simulink model "model_filters_bandpass"  (R2018a)
settings: Solver=VariableStepAuto  StartTime=0.0  StopTime=6  RelTol=1e-3
PreLoadFcn:
  | load('alberto_data.mat')
model workspace (MAT data in the model file):
  fc = Simulink.Parameter
  fc.Value = 10
  fc.DataType = 'auto'
  fc.Dimensions = [1 1]
undefined symbols (not defined in the file or in its folder): fc_2
libraries: dspmlti4 x1, dsparch4 x1
settings Model: Creator=stefanobuccelli  LastModifiedBy=stefanobuccelli

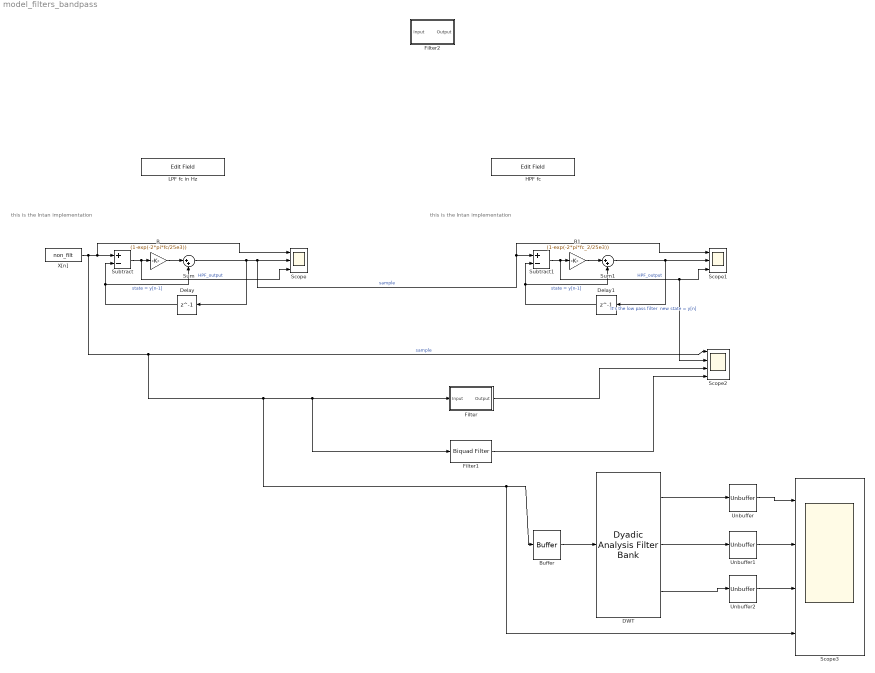
== system model_filters_bandpass ==
  note: this is the Intan implementation
  note: this is the Intan implementation
  B : Gain  Gain=(1-exp(-2*pi*fc/25e3))
  B1 : Gain  Gain=(1-exp(-2*pi*fc_2/25e3))
  Buffer : Buffer  OutputFrames=off
  DWT : dspmlti4/Dyadic Analysis Filter Bank  Wname=Biorthogonal  OrdRec_ordDec=[1 / 1]  Order=4  LPF="[0.0352   -0.0854   -0.1350   0.4599   0.8069   0.3327]"  HPF="[-0.3327    0.8069   -0.4599   -0.1350    0.0854    0.0352]"  NumLevels=2  tree=Asymmetric  Output=Multiple ports  OutputFrames=off
      settings: SourceProductName=DSP System Toolbox  SourceProductBaseCode=DS
  Delay : Delay  DelayLength=1
  Delay1 : Delay  DelayLength=1
  Filter : Subsystem  Tag=FilterWizardSubSystem
      settings: ErrorFcn=dspFilterRealizedInBasicElemsAlgLoopErrFcnCallback
  Filter1 : dsparch4/Biquad Filter  Tag=BlockMethodSubSystem  IIRFiltStruct=Direct form II  CoeffSource=Specify via dialog  BiQuadCoeffs=[1 0 -1 1 -1.99992831176449659 0.999934693355535975;1 0 -1 1 -1.99995897844210879 0.999961229592609468;1 0 -1 1 -1.9997987901469445 0.999805141210744264;1 0 -1 1 -1.99988145168083653 0.999883712729304319;1 0 -1 1 -1.99967234895056767 0.999678637128671221;1 0 -1 1 -1.99980407875227995 0.999806362624380718;1 0 -1 1 -1.99955099756990373 0.999557193946188249;1 0 -1 1 -1.99972693907547727 0.99972925660954115;1 0 -1 1 -1.99943663285096473 0.999442710022172998;1 0 -1 1 -1.99965016883954116 0.9996525313616208;1 0 -1 1 -1.99933100019716337 0.999336932639597553;1 0 -1 1 -1.99957397919015145 0.999576398765119833;1 0 -1 1 -1.9992355440381222 0.999241307193421191;1 0 -1 1 -1.99949878587869789 0.99950127682582135;1 0 -1 1 -1.99915183537296492 0.999157410502061416;1 0 -1 1 -1.99942476285883375 0.999427337308120389;1 0 -1 1 -1.99908090623175538 0.999086276782043647;1 0 -1 1 -1.99935249017064054 0.999355162168056532;1 0 -1 1 -1.99902340207156426 0.999028553701973743;1 0 -1 1 -1.9992827852671633 0.999285571050194887;1 0 -1 1 -1.99897998508968944 0.998984908853462139;1 0 -1 1 -1.99921628495669279 0.999219199786026469;1 0 -1 1 -1.99895111246551194 0.998955805384742823;1 0 -1 1 -1.99915365408997703 0.999156711568302991;1 0 -1 1 -1.99893596859811895 0.998940426918434321;1 0 -1 1 -1.99909664204870818 0.999099860745045421;1 0 -1 1 -1.99893512415378805 0.998939355238140814;1 0 -1 1 -1.99904541432707017 0.999048805016561126;1 0 -1 1 -1.99894631798573164 0.998950322878909391;1 0 -1 1 -1.99900276323179904 0.999006345900247505;1 0 -1 1 -1.99896927984751582 0.998973067828728856]  a0Flag=Warning  IC=0  ICnum=0  ICden=0  denAccumFracLength=30  denProdOutputFracLength=30  secondMemoryFracLength=15  roundingMode=Floor  overflowMode=off  ScaleValues=[0.000513716433989335787;0.000513716433989335787;0.000513689840814086441;0.000513689840814086441;0.000513663661699879275;0.000513663661699879275;0.000513638165030047425;0.000513638165030047425;0.000513613612073675926;0.000513613612073675926;0.000513590254319449798;0.000513590254319449798;0.000513568330913804225;0.000513568330913804225;0.000513548066228893744;0.000513548066228893744;0.000513529667584439208;0.000513529667584439208;0.00051351332314583881;0.00051351332314583881;0.000513499200019070586;0.000513499200019070586;0.000513487442560885479;0.000513487442560885479;0.000513478170920615164;0.000513478170920615164;0.000513471479827616378;0.000513471479827616378;0.000513467437635966185;0.000513467437635966185;0.000513466085635530317;1]  optimizeScaleValues=on  ScaleValueMode=Specify via input port (g)  scaleValueFracLength=14  FilterSource=Specify via dialog  FilterObject=BQF
      settings: SourceProductName=DSP System Toolbox
  Filter2 : Subsystem  Tag=FilterWizardSubSystem
      settings: ErrorFcn=dspFilterRealizedInBasicElemsAlgLoopErrFcnCallback
  HPF fc : EditField  WebBlockId=433  LabelPosition=Hide  Alignment=Center
  LPF fc in Hz : EditField  WebBlockId=206  LabelPosition=Hide  Alignment=Center
  Scope : Scope  NumInputPorts=3
  Scope1 : Scope  NumInputPorts=3
  Scope2 : Scope  NumInputPorts=4
  Scope3 : Scope  NumInputPorts=4
  Subtract : Sum  Inputs=+-
  Subtract1 : Sum  Inputs=+-
  Sum : Sum  Inputs=|++
  Sum1 : Sum  Inputs=|++
  Unbuffer : Unbuffer
  Unbuffer1 : Unbuffer
  Unbuffer2 : Unbuffer
  X[n] : FromWorkspace  VariableName=non_filt  SampleTime=1/25e3  OutputAfterFinalValue=Setting to zero
  wires:
  X[n]/1 -> Scope3/4, Buffer/1, Filter1/1, Filter/1(Input), Scope2/1, Scope/1, Subtract/1  "sample"
  Subtract/1 -> Scope/3, B/1  "HPF_output"
  B/1 -> Sum/1
  Delay/1 -> Sum/2, Subtract/2  "state = y[n-1]"
  Subtract1/1 -> Scope2/2, Scope1/3, B1/1  "HPF_output"
  B1/1 -> Sum1/1
  Delay1/1 -> Sum1/2, Subtract1/2  "state = y[n-1]"
  Sum1/1 -> Delay1/1, Scope1/2  "It's the low pass filter  new state = y[n]"
  Sum/1 -> Delay/1, Scope1/1, Subtract1/1, Scope/2  "sample"
  Filter/1(Output) -> Scope2/3
  Filter1/1 -> Scope2/4
  Buffer/1 -> DWT/1
  Unbuffer/1 -> Scope3/1
  Unbuffer1/1 -> Scope3/2
  Unbuffer2/1 -> Scope3/3
  DWT/2 -> Unbuffer1/1
  DWT/3 -> Unbuffer2/1
  DWT/1 -> Unbuffer/1

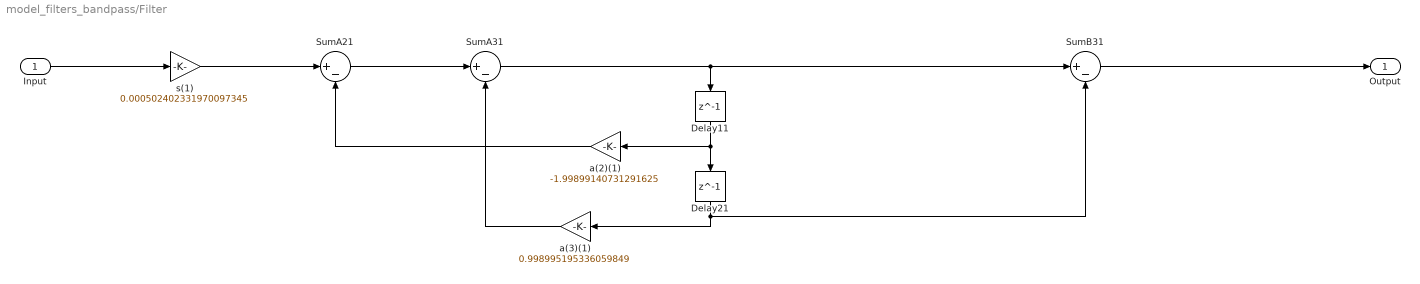
== system model_filters_bandpass/Filter ==
  Input : Inport
  Delay11 : Delay  DelayLength=1  InitialCondition=0
  Delay21 : Delay  DelayLength=1  InitialCondition=0
  SumA21 : Sum  Inputs=|+-  RndMeth=Nearest  SaturateOnIntegerOverflow=on  OutDataTypeStr=Inherit: Same as first input
  SumA31 : Sum  Inputs=|+-  RndMeth=Nearest  SaturateOnIntegerOverflow=on  OutDataTypeStr=Inherit: Same as first input
  SumB31 : Sum  Inputs=|+-  RndMeth=Nearest  SaturateOnIntegerOverflow=on  OutDataTypeStr=Inherit: Same as first input
  a(2)(1) : Gain  Gain=-1.99899140731291625  ParamDataTypeStr=double  RndMeth=Nearest  SaturateOnIntegerOverflow=on  OutDataTypeStr=Inherit: Same as input
  a(3)(1) : Gain  Gain=0.998995195336059849  ParamDataTypeStr=double  RndMeth=Nearest  SaturateOnIntegerOverflow=on  OutDataTypeStr=Inherit: Same as input
  s(1) : Gain  Gain=0.000502402331970097345  ParamDataTypeStr=double  RndMeth=Nearest  SaturateOnIntegerOverflow=on  OutDataTypeStr=Inherit: Same as input
  Output : Outport
  wires:
  Input/1 -> s(1)/1
  s(1)/1 -> SumA21/1
  SumA21/1 -> SumA31/1
  SumA31/1 -> SumB31/1, Delay11/1
  SumB31/1 -> Output/1
  a(2)(1)/1 -> SumA21/2
  Delay11/1 -> a(2)(1)/1, Delay21/1
  a(3)(1)/1 -> SumA31/2
  Delay21/1 -> a(3)(1)/1, SumB31/2

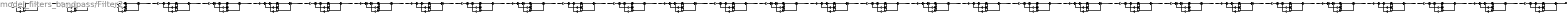
== system model_filters_bandpass/Filter2 ==
  Input : Inport
  Delay{11..19,21..29,110..131,210..231} (62 alike) : Delay  DelayLength=1  InitialCondition=0
  SumA{21..29,31..39,210..231,310..331} (62 alike) : Sum  Inputs=|+-  RndMeth=Nearest  SaturateOnIntegerOverflow=on  OutDataTypeStr=Inherit: Same as first input
  SumB{31..39,310..331} (31 alike) : Sum  Inputs=|+-  RndMeth=Nearest  SaturateOnIntegerOverflow=on  OutDataTypeStr=Inherit: Same as first input
  a(2)(1) : Gain  Gain=-1.99992831176449659  ParamDataTypeStr=double  RndMeth=Nearest  SaturateOnIntegerOverflow=on  OutDataTypeStr=Inherit: Same as input
  a(2)(10) : Gain  Gain=-1.99965016883954116  ParamDataTypeStr=double  RndMeth=Nearest  SaturateOnIntegerOverflow=on  OutDataTypeStr=Inherit: Same as input
  a(2)(11) : Gain  Gain=-1.99933100019716337  ParamDataTypeStr=double  RndMeth=Nearest  SaturateOnIntegerOverflow=on  OutDataTypeStr=Inherit: Same as input
  a(2)(12) : Gain  Gain=-1.99957397919015145  ParamDataTypeStr=double  RndMeth=Nearest  SaturateOnIntegerOverflow=on  OutDataTypeStr=Inherit: Same as input
  a(2)(13) : Gain  Gain=-1.9992355440381222  ParamDataTypeStr=double  RndMeth=Nearest  SaturateOnIntegerOverflow=on  OutDataTypeStr=Inherit: Same as input
  a(2)(14) : Gain  Gain=-1.99949878587869789  ParamDataTypeStr=double  RndMeth=Nearest  SaturateOnIntegerOverflow=on  OutDataTypeStr=Inherit: Same as input
  a(2)(15) : Gain  Gain=-1.99915183537296492  ParamDataTypeStr=double  RndMeth=Nearest  SaturateOnIntegerOverflow=on  OutDataTypeStr=Inherit: Same as input
  a(2)(16) : Gain  Gain=-1.99942476285883375  ParamDataTypeStr=double  RndMeth=Nearest  SaturateOnIntegerOverflow=on  OutDataTypeStr=Inherit: Same as input
  a(2)(17) : Gain  Gain=-1.99908090623175538  ParamDataTypeStr=double  RndMeth=Nearest  SaturateOnIntegerOverflow=on  OutDataTypeStr=Inherit: Same as input
  a(2)(18) : Gain  Gain=-1.99935249017064054  ParamDataTypeStr=double  RndMeth=Nearest  SaturateOnIntegerOverflow=on  OutDataTypeStr=Inherit: Same as input
  a(2)(19) : Gain  Gain=-1.99902340207156426  ParamDataTypeStr=double  RndMeth=Nearest  SaturateOnIntegerOverflow=on  OutDataTypeStr=Inherit: Same as input
  a(2)(2) : Gain  Gain=-1.99995897844210879  ParamDataTypeStr=double  RndMeth=Nearest  SaturateOnIntegerOverflow=on  OutDataTypeStr=Inherit: Same as input
  a(2)(20) : Gain  Gain=-1.9992827852671633  ParamDataTypeStr=double  RndMeth=Nearest  SaturateOnIntegerOverflow=on  OutDataTypeStr=Inherit: Same as input
  a(2)(21) : Gain  Gain=-1.99897998508968944  ParamDataTypeStr=double  RndMeth=Nearest  SaturateOnIntegerOverflow=on  OutDataTypeStr=Inherit: Same as input
  a(2)(22) : Gain  Gain=-1.99921628495669279  ParamDataTypeStr=double  RndMeth=Nearest  SaturateOnIntegerOverflow=on  OutDataTypeStr=Inherit: Same as input
  a(2)(23) : Gain  Gain=-1.99895111246551194  ParamDataTypeStr=double  RndMeth=Nearest  SaturateOnIntegerOverflow=on  OutDataTypeStr=Inherit: Same as input
  a(2)(24) : Gain  Gain=-1.99915365408997703  ParamDataTypeStr=double  RndMeth=Nearest  SaturateOnIntegerOverflow=on  OutDataTypeStr=Inherit: Same as input
  a(2)(25) : Gain  Gain=-1.99893596859811895  ParamDataTypeStr=double  RndMeth=Nearest  SaturateOnIntegerOverflow=on  OutDataTypeStr=Inherit: Same as input
  a(2)(26) : Gain  Gain=-1.99909664204870818  ParamDataTypeStr=double  RndMeth=Nearest  SaturateOnIntegerOverflow=on  OutDataTypeStr=Inherit: Same as input
  a(2)(27) : Gain  Gain=-1.99893512415378805  ParamDataTypeStr=double  RndMeth=Nearest  SaturateOnIntegerOverflow=on  OutDataTypeStr=Inherit: Same as input
  a(2)(28) : Gain  Gain=-1.99904541432707017  ParamDataTypeStr=double  RndMeth=Nearest  SaturateOnIntegerOverflow=on  OutDataTypeStr=Inherit: Same as input
  a(2)(29) : Gain  Gain=-1.99894631798573164  ParamDataTypeStr=double  RndMeth=Nearest  SaturateOnIntegerOverflow=on  OutDataTypeStr=Inherit: Same as input
  a(2)(3) : Gain  Gain=-1.9997987901469445  ParamDataTypeStr=double  RndMeth=Nearest  SaturateOnIntegerOverflow=on  OutDataTypeStr=Inherit: Same as input
  a(2)(30) : Gain  Gain=-1.99900276323179904  ParamDataTypeStr=double  RndMeth=Nearest  SaturateOnIntegerOverflow=on  OutDataTypeStr=Inherit: Same as input
  a(2)(31) : Gain  Gain=-1.99896927984751582  ParamDataTypeStr=double  RndMeth=Nearest  SaturateOnIntegerOverflow=on  OutDataTypeStr=Inherit: Same as input
  a(2)(4) : Gain  Gain=-1.99988145168083653  ParamDataTypeStr=double  RndMeth=Nearest  SaturateOnIntegerOverflow=on  OutDataTypeStr=Inherit: Same as input
  a(2)(5) : Gain  Gain=-1.99967234895056767  ParamDataTypeStr=double  RndMeth=Nearest  SaturateOnIntegerOverflow=on  OutDataTypeStr=Inherit: Same as input
  a(2)(6) : Gain  Gain=-1.99980407875227995  ParamDataTypeStr=double  RndMeth=Nearest  SaturateOnIntegerOverflow=on  OutDataTypeStr=Inherit: Same as input
  a(2)(7) : Gain  Gain=-1.99955099756990373  ParamDataTypeStr=double  RndMeth=Nearest  SaturateOnIntegerOverflow=on  OutDataTypeStr=Inherit: Same as input
  a(2)(8) : Gain  Gain=-1.99972693907547727  ParamDataTypeStr=double  RndMeth=Nearest  SaturateOnIntegerOverflow=on  OutDataTypeStr=Inherit: Same as input
  a(2)(9) : Gain  Gain=-1.99943663285096473  ParamDataTypeStr=double  RndMeth=Nearest  SaturateOnIntegerOverflow=on  OutDataTypeStr=Inherit: Same as input
  a(3)(1) : Gain  Gain=0.999934693355535975  ParamDataTypeStr=double  RndMeth=Nearest  SaturateOnIntegerOverflow=on  OutDataTypeStr=Inherit: Same as input
  a(3)(10) : Gain  Gain=0.9996525313616208  ParamDataTypeStr=double  RndMeth=Nearest  SaturateOnIntegerOverflow=on  OutDataTypeStr=Inherit: Same as input
  a(3)(11) : Gain  Gain=0.999336932639597553  ParamDataTypeStr=double  RndMeth=Nearest  SaturateOnIntegerOverflow=on  OutDataTypeStr=Inherit: Same as input
  a(3)(12) : Gain  Gain=0.999576398765119833  ParamDataTypeStr=double  RndMeth=Nearest  SaturateOnIntegerOverflow=on  OutDataTypeStr=Inherit: Same as input
  a(3)(13) : Gain  Gain=0.999241307193421191  ParamDataTypeStr=double  RndMeth=Nearest  SaturateOnIntegerOverflow=on  OutDataTypeStr=Inherit: Same as input
  a(3)(14) : Gain  Gain=0.99950127682582135  ParamDataTypeStr=double  RndMeth=Nearest  SaturateOnIntegerOverflow=on  OutDataTypeStr=Inherit: Same as input
  a(3)(15) : Gain  Gain=0.999157410502061416  ParamDataTypeStr=double  RndMeth=Nearest  SaturateOnIntegerOverflow=on  OutDataTypeStr=Inherit: Same as input
  a(3)(16) : Gain  Gain=0.999427337308120389  ParamDataTypeStr=double  RndMeth=Nearest  SaturateOnIntegerOverflow=on  OutDataTypeStr=Inherit: Same as input
  a(3)(17) : Gain  Gain=0.999086276782043647  ParamDataTypeStr=double  RndMeth=Nearest  SaturateOnIntegerOverflow=on  OutDataTypeStr=Inherit: Same as input
  a(3)(18) : Gain  Gain=0.999355162168056532  ParamDataTypeStr=double  RndMeth=Nearest  SaturateOnIntegerOverflow=on  OutDataTypeStr=Inherit: Same as input
  a(3)(19) : Gain  Gain=0.999028553701973743  ParamDataTypeStr=double  RndMeth=Nearest  SaturateOnIntegerOverflow=on  OutDataTypeStr=Inherit: Same as input
  a(3)(2) : Gain  Gain=0.999961229592609468  ParamDataTypeStr=double  RndMeth=Nearest  SaturateOnIntegerOverflow=on  OutDataTypeStr=Inherit: Same as input
  a(3)(20) : Gain  Gain=0.999285571050194887  ParamDataTypeStr=double  RndMeth=Nearest  SaturateOnIntegerOverflow=on  OutDataTypeStr=Inherit: Same as input
  a(3)(21) : Gain  Gain=0.998984908853462139  ParamDataTypeStr=double  RndMeth=Nearest  SaturateOnIntegerOverflow=on  OutDataTypeStr=Inherit: Same as input
  a(3)(22) : Gain  Gain=0.999219199786026469  ParamDataTypeStr=double  RndMeth=Nearest  SaturateOnIntegerOverflow=on  OutDataTypeStr=Inherit: Same as input
  a(3)(23) : Gain  Gain=0.998955805384742823  ParamDataTypeStr=double  RndMeth=Nearest  SaturateOnIntegerOverflow=on  OutDataTypeStr=Inherit: Same as input
  a(3)(24) : Gain  Gain=0.999156711568302991  ParamDataTypeStr=double  RndMeth=Nearest  SaturateOnIntegerOverflow=on  OutDataTypeStr=Inherit: Same as input
  a(3)(25) : Gain  Gain=0.998940426918434321  ParamDataTypeStr=double  RndMeth=Nearest  SaturateOnIntegerOverflow=on  OutDataTypeStr=Inherit: Same as input
  a(3)(26) : Gain  Gain=0.999099860745045421  ParamDataTypeStr=double  RndMeth=Nearest  SaturateOnIntegerOverflow=on  OutDataTypeStr=Inherit: Same as input
  a(3)(27) : Gain  Gain=0.998939355238140814  ParamDataTypeStr=double  RndMeth=Nearest  SaturateOnIntegerOverflow=on  OutDataTypeStr=Inherit: Same as input
  a(3)(28) : Gain  Gain=0.999048805016561126  ParamDataTypeStr=double  RndMeth=Nearest  SaturateOnIntegerOverflow=on  OutDataTypeStr=Inherit: Same as input
  a(3)(29) : Gain  Gain=0.998950322878909391  ParamDataTypeStr=double  RndMeth=Nearest  SaturateOnIntegerOverflow=on  OutDataTypeStr=Inherit: Same as input
  a(3)(3) : Gain  Gain=0.999805141210744264  ParamDataTypeStr=double  RndMeth=Nearest  SaturateOnIntegerOverflow=on  OutDataTypeStr=Inherit: Same as input
  a(3)(30) : Gain  Gain=0.999006345900247505  ParamDataTypeStr=double  RndMeth=Nearest  SaturateOnIntegerOverflow=on  OutDataTypeStr=Inherit: Same as input
  a(3)(31) : Gain  Gain=0.998973067828728856  ParamDataTypeStr=double  RndMeth=Nearest  SaturateOnIntegerOverflow=on  OutDataTypeStr=Inherit: Same as input
  a(3)(4) : Gain  Gain=0.999883712729304319  ParamDataTypeStr=double  RndMeth=Nearest  SaturateOnIntegerOverflow=on  OutDataTypeStr=Inherit: Same as input
  a(3)(5) : Gain  Gain=0.999678637128671221  ParamDataTypeStr=double  RndMeth=Nearest  SaturateOnIntegerOverflow=on  OutDataTypeStr=Inherit: Same as input
  a(3)(6) : Gain  Gain=0.999806362624380718  ParamDataTypeStr=double  RndMeth=Nearest  SaturateOnIntegerOverflow=on  OutDataTypeStr=Inherit: Same as input
  a(3)(7) : Gain  Gain=0.999557193946188249  ParamDataTypeStr=double  RndMeth=Nearest  SaturateOnIntegerOverflow=on  OutDataTypeStr=Inherit: Same as input
  a(3)(8) : Gain  Gain=0.99972925660954115  ParamDataTypeStr=double  RndMeth=Nearest  SaturateOnIntegerOverflow=on  OutDataTypeStr=Inherit: Same as input
  a(3)(9) : Gain  Gain=0.999442710022172998  ParamDataTypeStr=double  RndMeth=Nearest  SaturateOnIntegerOverflow=on  OutDataTypeStr=Inherit: Same as input
  s(1) : Gain  Gain=0.000513716433989335787  ParamDataTypeStr=double  RndMeth=Nearest  SaturateOnIntegerOverflow=on  OutDataTypeStr=Inherit: Same as input
  s(10) : Gain  Gain=0.000513613612073675926  ParamDataTypeStr=double  RndMeth=Nearest  SaturateOnIntegerOverflow=on  OutDataTypeStr=Inherit: Same as input
  s(11) : Gain  Gain=0.000513590254319449798  ParamDataTypeStr=double  RndMeth=Nearest  SaturateOnIntegerOverflow=on  OutDataTypeStr=Inherit: Same as input
  s(12) : Gain  Gain=0.000513590254319449798  ParamDataTypeStr=double  RndMeth=Nearest  SaturateOnIntegerOverflow=on  OutDataTypeStr=Inherit: Same as input
  s(13) : Gain  Gain=0.000513568330913804225  ParamDataTypeStr=double  RndMeth=Nearest  SaturateOnIntegerOverflow=on  OutDataTypeStr=Inherit: Same as input
  s(14) : Gain  Gain=0.000513568330913804225  ParamDataTypeStr=double  RndMeth=Nearest  SaturateOnIntegerOverflow=on  OutDataTypeStr=Inherit: Same as input
  s(15) : Gain  Gain=0.000513548066228893744  ParamDataTypeStr=double  RndMeth=Nearest  SaturateOnIntegerOverflow=on  OutDataTypeStr=Inherit: Same as input
  s(16) : Gain  Gain=0.000513548066228893744  ParamDataTypeStr=double  RndMeth=Nearest  SaturateOnIntegerOverflow=on  OutDataTypeStr=Inherit: Same as input
  s(17) : Gain  Gain=0.000513529667584439208  ParamDataTypeStr=double  RndMeth=Nearest  SaturateOnIntegerOverflow=on  OutDataTypeStr=Inherit: Same as input
  s(18) : Gain  Gain=0.000513529667584439208  ParamDataTypeStr=double  RndMeth=Nearest  SaturateOnIntegerOverflow=on  OutDataTypeStr=Inherit: Same as input
  s(19) : Gain  Gain=0.00051351332314583881  ParamDataTypeStr=double  RndMeth=Nearest  SaturateOnIntegerOverflow=on  OutDataTypeStr=Inherit: Same as input
  s(2) : Gain  Gain=0.000513716433989335787  ParamDataTypeStr=double  RndMeth=Nearest  SaturateOnIntegerOverflow=on  OutDataTypeStr=Inherit: Same as input
  s(20) : Gain  Gain=0.00051351332314583881  ParamDataTypeStr=double  RndMeth=Nearest  SaturateOnIntegerOverflow=on  OutDataTypeStr=Inherit: Same as input
  s(21) : Gain  Gain=0.000513499200019070586  ParamDataTypeStr=double  RndMeth=Nearest  SaturateOnIntegerOverflow=on  OutDataTypeStr=Inherit: Same as input
  s(22) : Gain  Gain=0.000513499200019070586  ParamDataTypeStr=double  RndMeth=Nearest  SaturateOnIntegerOverflow=on  OutDataTypeStr=Inherit: Same as input
  s(23) : Gain  Gain=0.000513487442560885479  ParamDataTypeStr=double  RndMeth=Nearest  SaturateOnIntegerOverflow=on  OutDataTypeStr=Inherit: Same as input
  s(24) : Gain  Gain=0.000513487442560885479  ParamDataTypeStr=double  RndMeth=Nearest  SaturateOnIntegerOverflow=on  OutDataTypeStr=Inherit: Same as input
  s(25) : Gain  Gain=0.000513478170920615164  ParamDataTypeStr=double  RndMeth=Nearest  SaturateOnIntegerOverflow=on  OutDataTypeStr=Inherit: Same as input
  s(26) : Gain  Gain=0.000513478170920615164  ParamDataTypeStr=double  RndMeth=Nearest  SaturateOnIntegerOverflow=on  OutDataTypeStr=Inherit: Same as input
  s(27) : Gain  Gain=0.000513471479827616378  ParamDataTypeStr=double  RndMeth=Nearest  SaturateOnIntegerOverflow=on  OutDataTypeStr=Inherit: Same as input
  s(28) : Gain  Gain=0.000513471479827616378  ParamDataTypeStr=double  RndMeth=Nearest  SaturateOnIntegerOverflow=on  OutDataTypeStr=Inherit: Same as input
  s(29) : Gain  Gain=0.000513467437635966185  ParamDataTypeStr=double  RndMeth=Nearest  SaturateOnIntegerOverflow=on  OutDataTypeStr=Inherit: Same as input
  s(3) : Gain  Gain=0.000513689840814086441  ParamDataTypeStr=double  RndMeth=Nearest  SaturateOnIntegerOverflow=on  OutDataTypeStr=Inherit: Same as input
  s(30) : Gain  Gain=0.000513467437635966185  ParamDataTypeStr=double  RndMeth=Nearest  SaturateOnIntegerOverflow=on  OutDataTypeStr=Inherit: Same as input
  s(31) : Gain  Gain=0.000513466085635530317  ParamDataTypeStr=double  RndMeth=Nearest  SaturateOnIntegerOverflow=on  OutDataTypeStr=Inherit: Same as input
  s(4) : Gain  Gain=0.000513689840814086441  ParamDataTypeStr=double  RndMeth=Nearest  SaturateOnIntegerOverflow=on  OutDataTypeStr=Inherit: Same as input
  s(5) : Gain  Gain=0.000513663661699879275  ParamDataTypeStr=double  RndMeth=Nearest  SaturateOnIntegerOverflow=on  OutDataTypeStr=Inherit: Same as input
  s(6) : Gain  Gain=0.000513663661699879275  ParamDataTypeStr=double  RndMeth=Nearest  SaturateOnIntegerOverflow=on  OutDataTypeStr=Inherit: Same as input
  s(7) : Gain  Gain=0.000513638165030047425  ParamDataTypeStr=double  RndMeth=Nearest  SaturateOnIntegerOverflow=on  OutDataTypeStr=Inherit: Same as input
  s(8) : Gain  Gain=0.000513638165030047425  ParamDataTypeStr=double  RndMeth=Nearest  SaturateOnIntegerOverflow=on  OutDataTypeStr=Inherit: Same as input
  s(9) : Gain  Gain=0.000513613612073675926  ParamDataTypeStr=double  RndMeth=Nearest  SaturateOnIntegerOverflow=on  OutDataTypeStr=Inherit: Same as input
  Output : Outport
  wires:
  Input/1 -> s(1)/1
  s(1)/1 -> SumA21/1
  SumA21/1 -> SumA31/1
  SumA31/1 -> SumB31/1, Delay11/1
  SumB31/1 -> [Sect1]
  a(2)(1)/1 -> SumA21/2
  Delay11/1 -> a(2)(1)/1, Delay21/1
  a(3)(1)/1 -> SumA31/2
  Delay21/1 -> a(3)(1)/1, SumB31/2
  [Sect1] -> s(2)/1
  s(2)/1 -> SumA22/1
  SumA22/1 -> SumA32/1
  SumA32/1 -> SumB32/1, Delay12/1
  SumB32/1 -> [Sect2]
  a(2)(2)/1 -> SumA22/2
  Delay12/1 -> a(2)(2)/1, Delay22/1
  a(3)(2)/1 -> SumA32/2
  Delay22/1 -> a(3)(2)/1, SumB32/2
  [Sect2] -> s(3)/1
  s(3)/1 -> SumA23/1
  SumA23/1 -> SumA33/1
  SumA33/1 -> SumB33/1, Delay13/1
  SumB33/1 -> [Sect3]
  a(2)(3)/1 -> SumA23/2
  Delay13/1 -> a(2)(3)/1, Delay23/1
  a(3)(3)/1 -> SumA33/2
  Delay23/1 -> a(3)(3)/1, SumB33/2
  [Sect3] -> s(4)/1
  s(4)/1 -> SumA24/1
  SumA24/1 -> SumA34/1
  SumA34/1 -> SumB34/1, Delay14/1
  SumB34/1 -> [Sect4]
  a(2)(4)/1 -> SumA24/2
  Delay14/1 -> a(2)(4)/1, Delay24/1
  a(3)(4)/1 -> SumA34/2
  Delay24/1 -> a(3)(4)/1, SumB34/2
  [Sect4] -> s(5)/1
  s(5)/1 -> SumA25/1
  SumA25/1 -> SumA35/1
  SumA35/1 -> SumB35/1, Delay15/1
  SumB35/1 -> [Sect5]
  a(2)(5)/1 -> SumA25/2
  Delay15/1 -> a(2)(5)/1, Delay25/1
  a(3)(5)/1 -> SumA35/2
  Delay25/1 -> a(3)(5)/1, SumB35/2
  [Sect5] -> s(6)/1
  s(6)/1 -> SumA26/1
  SumA26/1 -> SumA36/1
  SumA36/1 -> SumB36/1, Delay16/1
  SumB36/1 -> [Sect6]
  a(2)(6)/1 -> SumA26/2
  Delay16/1 -> a(2)(6)/1, Delay26/1
  a(3)(6)/1 -> SumA36/2
  Delay26/1 -> a(3)(6)/1, SumB36/2
  [Sect6] -> s(7)/1
  s(7)/1 -> SumA27/1
  SumA27/1 -> SumA37/1
  SumA37/1 -> SumB37/1, Delay17/1
  SumB37/1 -> [Sect7]
  a(2)(7)/1 -> SumA27/2
  Delay17/1 -> a(2)(7)/1, Delay27/1
  a(3)(7)/1 -> SumA37/2
  Delay27/1 -> a(3)(7)/1, SumB37/2
  [Sect7] -> s(8)/1
  s(8)/1 -> SumA28/1
  SumA28/1 -> SumA38/1
  SumA38/1 -> SumB38/1, Delay18/1
  SumB38/1 -> [Sect8]
  a(2)(8)/1 -> SumA28/2
  Delay18/1 -> a(2)(8)/1, Delay28/1
  a(3)(8)/1 -> SumA38/2
  Delay28/1 -> a(3)(8)/1, SumB38/2
  [Sect8] -> s(9)/1
  s(9)/1 -> SumA29/1
  SumA29/1 -> SumA39/1
  SumA39/1 -> SumB39/1, Delay19/1
  SumB39/1 -> [Sect9]
  a(2)(9)/1 -> SumA29/2
  Delay19/1 -> a(2)(9)/1, Delay29/1
  a(3)(9)/1 -> SumA39/2
  Delay29/1 -> a(3)(9)/1, SumB39/2
  [Sect9] -> s(10)/1
  s(10)/1 -> SumA210/1
  SumA210/1 -> SumA310/1
  SumA310/1 -> SumB310/1, Delay110/1
  SumB310/1 -> [Sect10]
  a(2)(10)/1 -> SumA210/2
  Delay110/1 -> a(2)(10)/1, Delay210/1
  a(3)(10)/1 -> SumA310/2
  Delay210/1 -> a(3)(10)/1, SumB310/2
  [Sect10] -> s(11)/1
  s(11)/1 -> SumA211/1
  SumA211/1 -> SumA311/1
  SumA311/1 -> SumB311/1, Delay111/1
  SumB311/1 -> [Sect11]
  a(2)(11)/1 -> SumA211/2
  Delay111/1 -> a(2)(11)/1, Delay211/1
  a(3)(11)/1 -> SumA311/2
  Delay211/1 -> a(3)(11)/1, SumB311/2
  [Sect11] -> s(12)/1
  s(12)/1 -> SumA212/1
  SumA212/1 -> SumA312/1
  SumA312/1 -> SumB312/1, Delay112/1
  SumB312/1 -> [Sect12]
  a(2)(12)/1 -> SumA212/2
  Delay112/1 -> a(2)(12)/1, Delay212/1
  a(3)(12)/1 -> SumA312/2
  Delay212/1 -> a(3)(12)/1, SumB312/2
  [Sect12] -> s(13)/1
  s(13)/1 -> SumA213/1
  SumA213/1 -> SumA313/1
  SumA313/1 -> SumB313/1, Delay113/1
  SumB313/1 -> [Sect13]
  a(2)(13)/1 -> SumA213/2
  Delay113/1 -> a(2)(13)/1, Delay213/1
  a(3)(13)/1 -> SumA313/2
  Delay213/1 -> a(3)(13)/1, SumB313/2
  [Sect13] -> s(14)/1
  s(14)/1 -> SumA214/1
  SumA214/1 -> SumA314/1
  SumA314/1 -> SumB314/1, Delay114/1
  SumB314/1 -> [Sect14]
  a(2)(14)/1 -> SumA214/2
  Delay114/1 -> a(2)(14)/1, Delay214/1
  a(3)(14)/1 -> SumA314/2
  Delay214/1 -> a(3)(14)/1, SumB314/2
  [Sect14] -> s(15)/1
  s(15)/1 -> SumA215/1
  SumA215/1 -> SumA315/1
  SumA315/1 -> SumB315/1, Delay115/1
  SumB315/1 -> [Sect15]
  a(2)(15)/1 -> SumA215/2
  Delay115/1 -> a(2)(15)/1, Delay215/1
  a(3)(15)/1 -> SumA315/2
  Delay215/1 -> a(3)(15)/1, SumB315/2
  [Sect15] -> s(16)/1
  s(16)/1 -> SumA216/1
  SumA216/1 -> SumA316/1
  SumA316/1 -> SumB316/1, Delay116/1
  SumB316/1 -> [Sect16]
  a(2)(16)/1 -> SumA216/2
  Delay116/1 -> a(2)(16)/1, Delay216/1
  a(3)(16)/1 -> SumA316/2
  Delay216/1 -> a(3)(16)/1, SumB316/2
  [Sect16] -> s(17)/1
  s(17)/1 -> SumA217/1
  SumA217/1 -> SumA317/1
  SumA317/1 -> SumB317/1, Delay117/1
  SumB317/1 -> [Sect17]
  a(2)(17)/1 -> SumA217/2
  Delay117/1 -> a(2)(17)/1, Delay217/1
  a(3)(17)/1 -> SumA317/2
  Delay217/1 -> a(3)(17)/1, SumB317/2
  [Sect17] -> s(18)/1
  s(18)/1 -> SumA218/1
  SumA218/1 -> SumA318/1
  SumA318/1 -> SumB318/1, Delay118/1
  SumB318/1 -> [Sect18]
  a(2)(18)/1 -> SumA218/2
  Delay118/1 -> a(2)(18)/1, Delay218/1
  a(3)(18)/1 -> SumA318/2
  Delay218/1 -> a(3)(18)/1, SumB318/2
  [Sect18] -> s(19)/1
  s(19)/1 -> SumA219/1
  SumA219/1 -> SumA319/1
  SumA319/1 -> SumB319/1, Delay119/1
  SumB319/1 -> [Sect19]
  a(2)(19)/1 -> SumA219/2
  Delay119/1 -> a(2)(19)/1, Delay219/1
  a(3)(19)/1 -> SumA319/2
  Delay219/1 -> a(3)(19)/1, SumB319/2
  [Sect19] -> s(20)/1
  s(20)/1 -> SumA220/1
  SumA220/1 -> SumA320/1
  SumA320/1 -> SumB320/1, Delay120/1
  SumB320/1 -> [Sect20]
  a(2)(20)/1 -> SumA220/2
  Delay120/1 -> a(2)(20)/1, Delay220/1
  a(3)(20)/1 -> SumA320/2
  Delay220/1 -> a(3)(20)/1, SumB320/2
  [Sect20] -> s(21)/1
  s(21)/1 -> SumA221/1
  SumA221/1 -> SumA321/1
  SumA321/1 -> SumB321/1, Delay121/1
  SumB321/1 -> [Sect21]
  a(2)(21)/1 -> SumA221/2
  Delay121/1 -> a(2)(21)/1, Delay221/1
  a(3)(21)/1 -> SumA321/2
  Delay221/1 -> a(3)(21)/1, SumB321/2
  [Sect21] -> s(22)/1
  s(22)/1 -> SumA222/1
  SumA222/1 -> SumA322/1
  SumA322/1 -> SumB322/1, Delay122/1
  SumB322/1 -> [Sect22]
  a(2)(22)/1 -> SumA222/2
  Delay122/1 -> a(2)(22)/1, Delay222/1
  a(3)(22)/1 -> SumA322/2
  Delay222/1 -> a(3)(22)/1, SumB322/2
  [Sect22] -> s(23)/1
  s(23)/1 -> SumA223/1
  SumA223/1 -> SumA323/1
  SumA323/1 -> SumB323/1, Delay123/1
  SumB323/1 -> [Sect23]
  a(2)(23)/1 -> SumA223/2
  Delay123/1 -> a(2)(23)/1, Delay223/1
  a(3)(23)/1 -> SumA323/2
  Delay223/1 -> a(3)(23)/1, SumB323/2
  [Sect23] -> s(24)/1
  s(24)/1 -> SumA224/1
  SumA224/1 -> SumA324/1
  SumA324/1 -> SumB324/1, Delay124/1
  SumB324/1 -> [Sect24]
  a(2)(24)/1 -> SumA224/2
  Delay124/1 -> a(2)(24)/1, Delay224/1
  a(3)(24)/1 -> SumA324/2
  Delay224/1 -> a(3)(24)/1, SumB324/2
  [Sect24] -> s(25)/1
  s(25)/1 -> SumA225/1
  SumA225/1 -> SumA325/1
  SumA325/1 -> SumB325/1, Delay125/1
  SumB325/1 -> [Sect25]
  a(2)(25)/1 -> SumA225/2
  Delay125/1 -> a(2)(25)/1, Delay225/1
  a(3)(25)/1 -> SumA325/2
  Delay225/1 -> a(3)(25)/1, SumB325/2
  [Sect25] -> s(26)/1
  s(26)/1 -> SumA226/1
  SumA226/1 -> SumA326/1
  SumA326/1 -> SumB326/1, Delay126/1
  SumB326/1 -> [Sect26]
  a(2)(26)/1 -> SumA226/2
  Delay126/1 -> a(2)(26)/1, Delay226/1
  a(3)(26)/1 -> SumA326/2
  Delay226/1 -> a(3)(26)/1, SumB326/2
  [Sect26] -> s(27)/1
  s(27)/1 -> SumA227/1
  SumA227/1 -> SumA327/1
  SumA327/1 -> SumB327/1, Delay127/1
  SumB327/1 -> [Sect27]
  a(2)(27)/1 -> SumA227/2
  Delay127/1 -> a(2)(27)/1, Delay227/1
  a(3)(27)/1 -> SumA327/2
  Delay227/1 -> a(3)(27)/1, SumB327/2
  [Sect27] -> s(28)/1
  s(28)/1 -> SumA228/1
  SumA228/1 -> SumA328/1
  SumA328/1 -> SumB328/1, Delay128/1
  SumB328/1 -> [Sect28]
  a(2)(28)/1 -> SumA228/2
  Delay128/1 -> a(2)(28)/1, Delay228/1
  a(3)(28)/1 -> SumA328/2
  Delay228/1 -> a(3)(28)/1, SumB328/2
  [Sect28] -> s(29)/1
  s(29)/1 -> SumA229/1
  SumA229/1 -> SumA329/1
  SumA329/1 -> SumB329/1, Delay129/1
  SumB329/1 -> [Sect29]
  a(2)(29)/1 -> SumA229/2
  Delay129/1 -> a(2)(29)/1, Delay229/1
  a(3)(29)/1 -> SumA329/2
  Delay229/1 -> a(3)(29)/1, SumB329/2
  [Sect29] -> s(30)/1
  s(30)/1 -> SumA230/1
  SumA230/1 -> SumA330/1
  SumA330/1 -> SumB330/1, Delay130/1
  SumB330/1 -> [Sect30]
  a(2)(30)/1 -> SumA230/2
  Delay130/1 -> a(2)(30)/1, Delay230/1
  a(3)(30)/1 -> SumA330/2
  Delay230/1 -> a(3)(30)/1, SumB330/2
  [Sect30] -> s(31)/1
  s(31)/1 -> SumA231/1
  SumA231/1 -> SumA331/1
  SumA331/1 -> SumB331/1, Delay131/1
  SumB331/1 -> Output/1
  a(2)(31)/1 -> SumA231/2
  Delay131/1 -> a(2)(31)/1, Delay231/1
  a(3)(31)/1 -> SumA331/2
  Delay231/1 -> a(3)(31)/1, SumB331/2
